simulink model "bal_main_alpha"  (R2015a)
settings: Solver=ode45  StartTime=0.0  StopTime=600  RelTol=1e-3
undefined symbols (not defined in the file): Alfa_zad, Cxa_Delta_1, Cxa_Delta_2, Cxa_Delta_3, Cxa_pol, Cya_Delta_1, Cya_Delta_2, Cya_Delta_3, Cya_pol, Delta_1_zad, Delta_2_zad, Delta_3_zad, h_zad, h_zad_D1_D2, h_zad_D3, mz_Alfa, mz_Delta_1, mz_Delta_2, mz_Delta_3, xt_zad
libraries: simulink x5
settings Model: Creator=Admin  LastModifiedBy=гена

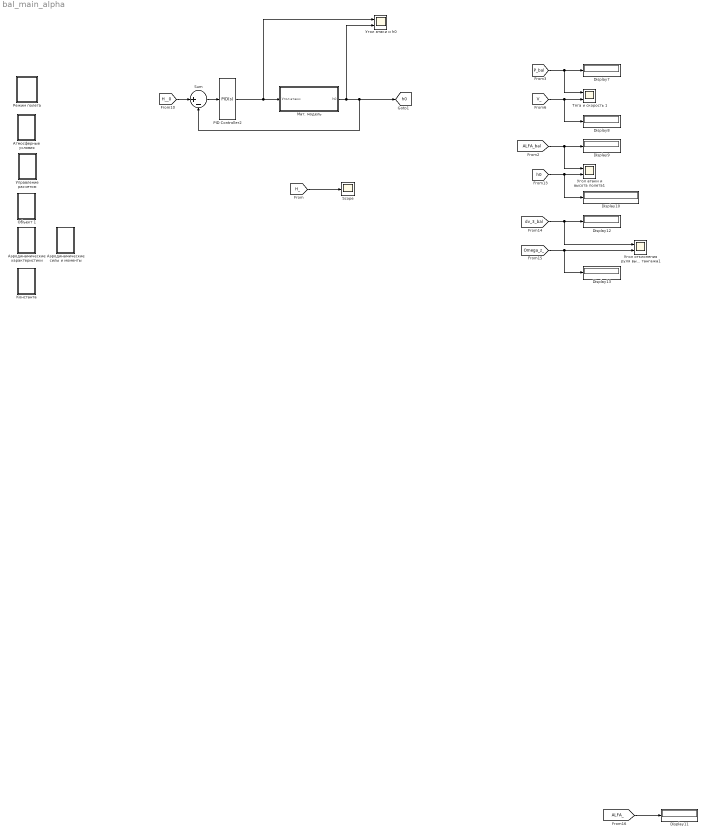
== system bal_main_alpha ==
  Display{7..13} (7 alike) : Display
  PID Controller2 : simulink/Continuous/PID Controller  Controller=PID  TimeDomain=Continuous-time  SampleTime=-1  IntegratorMethod=Forward Euler  FilterMethod=Forward Euler  Form=Parallel  UseFilter=on  ControllerParametersSource=internal  P=1.12  I=2  D=1  N=1  InitialConditionSource=internal  InitialConditionForIntegrator=0  InitialConditionForFilter=0  ExternalReset=none  LimitOutput=off  UpperSaturationLimit=inf  LowerSaturationLimit=-inf  LinearizeAsGain=on  AntiWindupMode=none  Kb=1  TrackingMode=off  Kt=1  PParamMin=[]  PParamMax=[]  IParamMin=[]  IParamMax=[]  DParamMin=[]  DParamMax=[]  NParamMin=[]  NParamMax=[]  KbParamMin=[]  KbParamMax=[]  KtParamMin=[]  KtParamMax=[]  POutMin=[]  POutMax=[]  IOutMin=[]  IOutMax=[]  DOutMin=[]  DOutMax=[]  NOutMin=[]  NOutMax=[]  KbOutMin=[]  KbOutMax=[]  KtOutMin=[]  KtOutMax=[]  IntegratorOutMin=[]  IntegratorOutMax=[]  FilterOutMin=[]  FilterOutMax=[]  SumOutMin=[]  SumOutMax=[]  SumI1OutMin=[]  SumI1OutMax=[]  SumI2OutMin=[]  SumI2OutMax=[]  SumI3OutMin=[]  SumI3OutMax=[]  SumDOutMin=[]  SumDOutMax=[]  SaturationOutMin=[]  SaturationOutMax=[]  IntegratorContinuousStateAttributes=''  IntegratorStateMustResolveToSignalObject=off  IntegratorRTWStateStorageClass=Auto  FilterContinuousStateAttributes=''  FilterStateMustResolveToSignalObject=off  FilterRTWStateStorageClass=Auto  DifferentiatorICPrevScaledInput=0  DifferentiatorOutMin=[]  DifferentiatorOutMax=[]
  Scope : Scope
  Sum : Sum  Inputs=|+-
  Атмосферные условия : Subsystem
  Аэродинамические характеристики : Subsystem
  Аэродинамические силы и моменты : Subsystem
  Константа : Subsystem
  Мат. модель : Subsystem
  Объект 1 : Subsystem
  Режим полета : Subsystem  mask(Параметры исходного полета){M_LA=1000, V_0=50, H_0=0.15}
      mask prompts: M_LA "Полетная масса, кг"; V_0 "Скорость полета, м/с"; H_0 "Высота полета, м"
  Тяга и скорость 1 : Scope  NumInputPorts=2
      settings: TimeRange=100  YMin=0~20  YMax=7000~55  SaveName=ScopeData3
  Угол атаки и высота полета1 : Scope  NumInputPorts=2
      settings: TimeRange=100  YMin=-5~-0.6000000000000001  YMax=20~0.2999999999999999  SaveName=ScopeData4
  Угол атаки и h0 : Scope  NumInputPorts=2
      settings: TimeRange=100  YMin=0~20  YMax=7000~55
  Угол отклонения руля высоты и угловая скорость тангажа1 : Scope  NumInputPorts=2
      settings: TimeRange=100  YMin=-6~-5  YMax=14~5  SaveName=ScopeData5
  Управление расчетом : Subsystem
  tag scope: h0=global
  wires:
  [P_bal] -> Display7/1, Тяга и скорость 1/1
  [V_] -> Display8/1, Тяга и скорость 1/2
  [ALFA_bal] -> Display9/1, Угол атаки и высота полета1/1
  [h0] -> Display10/1, Угол атаки и высота полета1/2
  [dv_3_bal] -> Display12/1, Угол отклонения руля высоты и угловая скорость тангажа1/1
  [Omega_z_] -> Display13/1, Угол отклонения руля высоты и угловая скорость тангажа1/2
  [ALFA_] -> Display11/1
  Sum/1 -> PID Controller2/1
  [H__0] -> Sum/1
  PID Controller2/1 -> Мат. модель/1(Угол атаки), Угол атаки и h0/1
  Мат. модель/1(h0) -> Угол атаки и h0/2, Sum/2, [h0]
  [H_] -> Scope/1

== system bal_main_alpha/Атмосферные условия ==
  Плотность : Constant  Value=1.225
  tag scope: Ro=global
  wires:
  Плотность/1 -> [Ro]

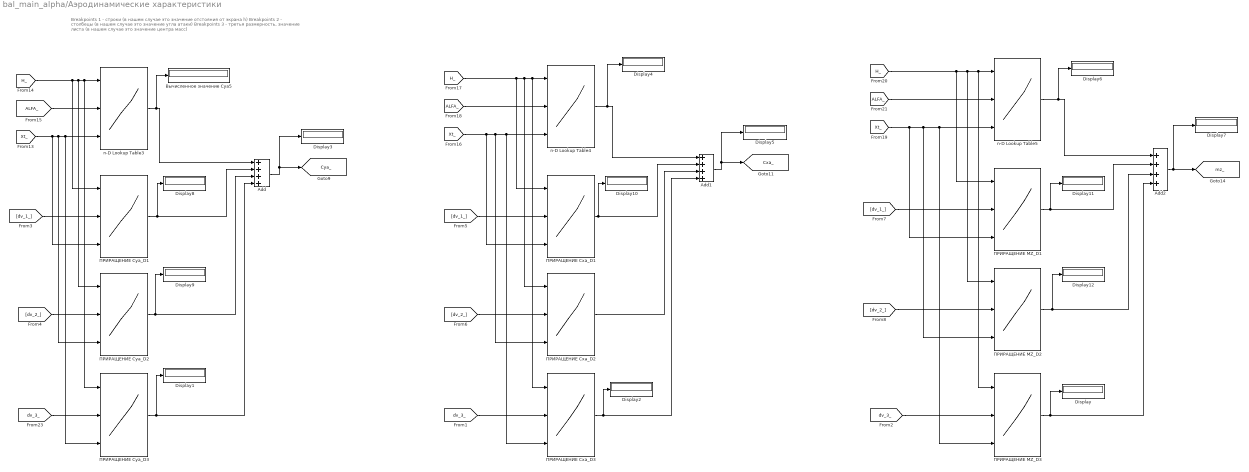
== system bal_main_alpha/Аэродинамические характеристики ==
  note: Breakpoints 1 - строки (в нашем случае это значение отстояния от экрана h)
      | Breakpoints 2 - столбецы (в нашем случае это значение угла атаки)
      | Breakpoints 3 - третья размерность, значение листа (в нашем случае это значение центра масс)
  Add : Sum  Inputs=++++
  Add1 : Sum  Inputs=++++
  Add2 : Sum  Inputs=++++
  Display{,1..12} (13 alike) : Display
  n-D Lookup Table3 : Lookup_n-D  NumberOfTableDimensions=3  BreakpointsForDimension1=h_zad  BreakpointsForDimension2=Alfa_zad  BreakpointsForDimension3=xt_zad  Table=Cya_pol  InternalRulePriority=Speed  RndMeth=Simplest  InputSameDT=on
  n-D Lookup Table4 : Lookup_n-D  NumberOfTableDimensions=3  BreakpointsForDimension1=h_zad  BreakpointsForDimension2=Alfa_zad  BreakpointsForDimension3=xt_zad  Table=Cxa_pol  InternalRulePriority=Speed  RndMeth=Simplest  InputSameDT=on
  n-D Lookup Table5 : Lookup_n-D  NumberOfTableDimensions=3  BreakpointsForDimension1=h_zad  BreakpointsForDimension2=Alfa_zad  BreakpointsForDimension3=xt_zad  Table=mz_Alfa  InternalRulePriority=Speed  RndMeth=Simplest  InputSameDT=on
  Вычисленное значение Суа5 : Display
  ПРИРАЩЕНИЕ Cxa_D1 : Lookup_n-D  NumberOfTableDimensions=3  BreakpointsForDimension1=h_zad_D1_D2  BreakpointsForDimension2=Delta_1_zad  BreakpointsForDimension3=xt_zad  Table=Cxa_Delta_1  InternalRulePriority=Speed  RndMeth=Simplest  InputSameDT=on
  ПРИРАЩЕНИЕ Cxa_D2 : Lookup_n-D  NumberOfTableDimensions=3  BreakpointsForDimension1=h_zad_D1_D2  BreakpointsForDimension2=Delta_2_zad  BreakpointsForDimension3=xt_zad  Table=Cxa_Delta_2  InternalRulePriority=Speed  RndMeth=Simplest  InputSameDT=on
  ПРИРАЩЕНИЕ Cxa_D3 : Lookup_n-D  NumberOfTableDimensions=3  BreakpointsForDimension1=h_zad_D3  BreakpointsForDimension2=Delta_3_zad  BreakpointsForDimension3=xt_zad  Table=Cxa_Delta_3  InternalRulePriority=Speed  RndMeth=Simplest  InputSameDT=on
  ПРИРАЩЕНИЕ Cya_D1 : Lookup_n-D  NumberOfTableDimensions=3  BreakpointsForDimension1=h_zad_D1_D2  BreakpointsForDimension2=Delta_1_zad  BreakpointsForDimension3=xt_zad  Table=Cya_Delta_1  InternalRulePriority=Speed  RndMeth=Simplest  InputSameDT=on
  ПРИРАЩЕНИЕ Cya_D2 : Lookup_n-D  NumberOfTableDimensions=3  BreakpointsForDimension1=h_zad_D1_D2  BreakpointsForDimension2=Delta_2_zad  BreakpointsForDimension3=xt_zad  Table=Cya_Delta_2  InternalRulePriority=Speed  RndMeth=Simplest  InputSameDT=on
  ПРИРАЩЕНИЕ Cya_D3 : Lookup_n-D  NumberOfTableDimensions=3  BreakpointsForDimension1=h_zad_D3  BreakpointsForDimension2=Delta_3_zad  BreakpointsForDimension3=xt_zad  Table=Cya_Delta_3  InternalRulePriority=Speed  RndMeth=Simplest  InputSameDT=on
  ПРИРАЩЕНИЕ MZ_D1 : Lookup_n-D  NumberOfTableDimensions=3  BreakpointsForDimension1=h_zad_D1_D2  BreakpointsForDimension2=Delta_1_zad  BreakpointsForDimension3=xt_zad  Table=mz_Delta_1  InternalRulePriority=Speed  RndMeth=Simplest  InputSameDT=on
  ПРИРАЩЕНИЕ MZ_D2 : Lookup_n-D  NumberOfTableDimensions=3  BreakpointsForDimension1=h_zad_D1_D2  BreakpointsForDimension2=Delta_2_zad  BreakpointsForDimension3=xt_zad  Table=mz_Delta_2  InternalRulePriority=Speed  RndMeth=Simplest  InputSameDT=on
  ПРИРАЩЕНИЕ MZ_D3 : Lookup_n-D  NumberOfTableDimensions=3  BreakpointsForDimension1=h_zad_D3  BreakpointsForDimension2=Delta_3_zad  BreakpointsForDimension3=xt_zad  Table=mz_Delta_3  InternalRulePriority=Speed  RndMeth=Simplest  InputSameDT=on
  tag scope: Cxa_=global, Cya_=global, mz_=global
  wires:
  [H_] -> ПРИРАЩЕНИЕ Cya_D3/1, n-D Lookup Table3/1, ПРИРАЩЕНИЕ Cya_D2/1, ПРИРАЩЕНИЕ Cya_D1/1
  [Xt_] -> ПРИРАЩЕНИЕ Cya_D2/3, ПРИРАЩЕНИЕ Cya_D3/3, n-D Lookup Table3/3, ПРИРАЩЕНИЕ Cya_D1/3
  n-D Lookup Table3/1 -> Вычисленное значение Суа5/1, Add/1
  [H_] -> ПРИРАЩЕНИЕ Cxa_D1/1, ПРИРАЩЕНИЕ Cxa_D2/1, ПРИРАЩЕНИЕ Cxa_D3/1, n-D Lookup Table4/1
  [Xt_] -> ПРИРАЩЕНИЕ Cxa_D1/3, ПРИРАЩЕНИЕ Cxa_D2/3, n-D Lookup Table4/3, ПРИРАЩЕНИЕ Cxa_D3/3
  [ALFA_] -> n-D Lookup Table5/2
  [ALFA_] -> n-D Lookup Table4/2
  [ALFA_] -> n-D Lookup Table3/2
  [Xt_] -> ПРИРАЩЕНИЕ MZ_D1/3, ПРИРАЩЕНИЕ MZ_D2/3, n-D Lookup Table5/3, ПРИРАЩЕНИЕ MZ_D3/3
  [dv_3_] -> ПРИРАЩЕНИЕ Cxa_D3/2
  Add/1 -> Display3/1, [Cya_]
  n-D Lookup Table4/1 -> Display4/1, Add1/1
  Add1/1 -> Display5/1, [Cxa_]
  n-D Lookup Table5/1 -> Display6/1, Add2/1
  Add2/1 -> Display7/1, [mz_]
  [dv_3_] -> ПРИРАЩЕНИЕ MZ_D3/2
  [dv_1_] -> ПРИРАЩЕНИЕ Cya_D1/2
  [dv_2_] -> ПРИРАЩЕНИЕ Cya_D2/2
  ПРИРАЩЕНИЕ Cya_D1/1 -> Display8/1, Add/2
  ПРИРАЩЕНИЕ Cya_D2/1 -> Display9/1, Add/3
  [dv_3_] -> ПРИРАЩЕНИЕ Cya_D3/2
  ПРИРАЩЕНИЕ Cya_D3/1 -> Display1/1, Add/4
  ПРИРАЩЕНИЕ Cxa_D3/1 -> Display2/1, Add1/4
  [dv_1_] -> ПРИРАЩЕНИЕ Cxa_D1/2
  ПРИРАЩЕНИЕ Cxa_D1/1 -> Display10/1, Add1/2
  [dv_2_] -> ПРИРАЩЕНИЕ Cxa_D2/2
  ПРИРАЩЕНИЕ Cxa_D2/1 -> Add1/3
  ПРИРАЩЕНИЕ MZ_D3/1 -> Display/1, Add2/4
  [dv_1_] -> ПРИРАЩЕНИЕ MZ_D1/2
  ПРИРАЩЕНИЕ MZ_D1/1 -> Display11/1, Add2/2
  [H_] -> ПРИРАЩЕНИЕ MZ_D2/1, ПРИРАЩЕНИЕ MZ_D3/1, n-D Lookup Table5/1, ПРИРАЩЕНИЕ MZ_D1/1
  [dv_2_] -> ПРИРАЩЕНИЕ MZ_D2/2
  ПРИРАЩЕНИЕ MZ_D2/1 -> Display12/1, Add2/3

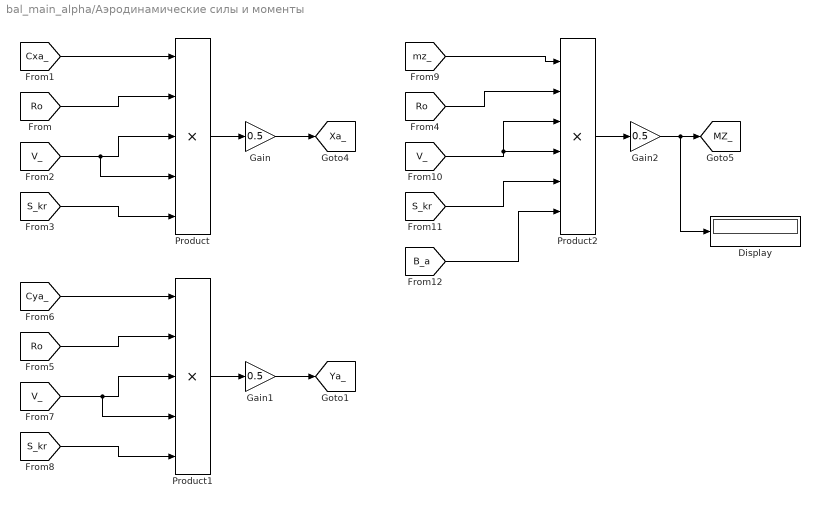
== system bal_main_alpha/Аэродинамические силы и моменты ==
  Display : Display
  Gain : Gain  Gain=0.5
  Gain1 : Gain  Gain=0.5
  Gain2 : Gain  Gain=0.5
  Product : Product  Inputs=*****
  Product1 : Product  Inputs=*****
  Product2 : Product  Inputs=******
  tag scope: MZ_=global, Xa_=global, Ya_=global
  wires:
  Product/1 -> Gain/1
  [S_kr] -> Product/5
  Gain/1 -> [Xa_]
  [Cxa_] -> Product/1
  [Ro] -> Product/2
  [V_] -> Product/4, Product/3
  Product1/1 -> Gain1/1
  [S_kr] -> Product1/5
  Gain1/1 -> [Ya_]
  [Cya_] -> Product1/1
  [Ro] -> Product1/2
  [V_] -> Product1/4, Product1/3
  Product2/1 -> Gain2/1
  [S_kr] -> Product2/5
  Gain2/1 -> Display/1, [MZ_]
  [mz_] -> Product2/1
  [Ro] -> Product2/2
  [B_a] -> Product2/6
  [V_] -> Product2/4, Product2/3

== system bal_main_alpha/Константа ==
  RAD : Constant  Value=57.3
  g : Constant  Value=9.81
  tag scope: RAD=global, g_=global
  wires:
  g/1 -> [g_]
  RAD/1 -> [RAD]

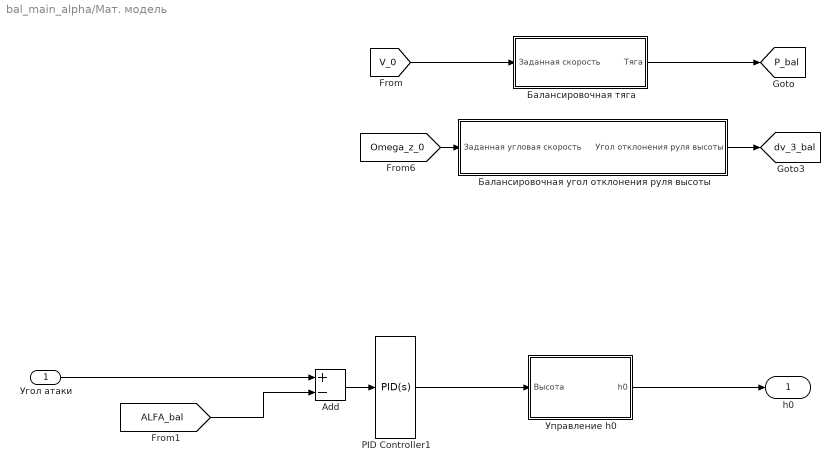
== system bal_main_alpha/Мат. модель ==
  Угол атаки : Inport
  Add : Sum  Inputs=+-
  PID Controller1 : simulink/Continuous/PID Controller  Controller=PID  TimeDomain=Continuous-time  SampleTime=-1  IntegratorMethod=Forward Euler  FilterMethod=Forward Euler  Form=Parallel  UseFilter=on  ControllerParametersSource=internal  P=0.0917439667717994  I=0.0166206189219194  D=-0.151733255398007  N=0.604639810377417  InitialConditionSource=internal  InitialConditionForIntegrator=0  InitialConditionForFilter=0  ExternalReset=none  LimitOutput=off  UpperSaturationLimit=inf  LowerSaturationLimit=-inf  LinearizeAsGain=on  AntiWindupMode=none  Kb=1  TrackingMode=off  Kt=1  PParamMin=[]  PParamMax=[]  IParamMin=[]  IParamMax=[]  DParamMin=[]  DParamMax=[]  NParamMin=[]  NParamMax=[]  KbParamMin=[]  KbParamMax=[]  KtParamMin=[]  KtParamMax=[]  POutMin=[]  POutMax=[]  IOutMin=[]  IOutMax=[]  DOutMin=[]  DOutMax=[]  NOutMin=[]  NOutMax=[]  KbOutMin=[]  KbOutMax=[]  KtOutMin=[]  KtOutMax=[]  IntegratorOutMin=[]  IntegratorOutMax=[]  FilterOutMin=[]  FilterOutMax=[]  SumOutMin=[]  SumOutMax=[]  SumI1OutMin=[]  SumI1OutMax=[]  SumI2OutMin=[]  SumI2OutMax=[]  SumI3OutMin=[]  SumI3OutMax=[]  SumDOutMin=[]  SumDOutMax=[]  SaturationOutMin=[]  SaturationOutMax=[]  IntegratorContinuousStateAttributes=''  IntegratorStateMustResolveToSignalObject=off  IntegratorRTWStateStorageClass=Auto  FilterContinuousStateAttributes=''  FilterStateMustResolveToSignalObject=off  FilterRTWStateStorageClass=Auto  DifferentiatorICPrevScaledInput=0  DifferentiatorOutMin=[]  DifferentiatorOutMax=[]
  Балансировочная угол отклонения руля высоты : Subsystem
  Балансировочная тяга : Subsystem
  Управление h0 : Subsystem
  h0 : Outport
  tag scope: P_bal=global, dv_3_bal=global
  wires:
  [V_0] -> Балансировочная тяга/1(Заданная скорость)
  [Omega_z_0] -> Балансировочная угол отклонения руля высоты/1(Заданная угловая скорость)
  Балансировочная угол отклонения руля высоты/1(Угол отклонения руля высоты) -> [dv_3_bal]
  Балансировочная тяга/1(Тяга) -> [P_bal]
  Add/1 -> PID Controller1/1
  Угол атаки/1 -> Add/1
  [ALFA_bal] -> Add/2
  PID Controller1/1 -> Управление h0/1(Высота)
  Управление h0/1(h0) -> h0/1

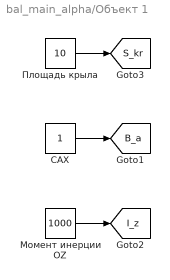
== system bal_main_alpha/Объект 1 ==
  Момент инерции ОZ : Constant  Value=1000
  Площадь крыла : Constant  Value=10
  САХ : Constant
  tag scope: B_a=global, I_z=global, S_kr=global
  wires:
  Площадь крыла/1 -> [S_kr]
  САХ/1 -> [B_a]
  Момент инерции ОZ/1 -> [I_z]

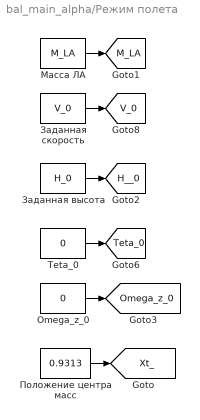
== system bal_main_alpha/Режим полета ==
  Omega_z_0 : Constant  Value=0
  Teta_0 : Constant  Value=0
  Заданная высота : Constant  Value=H_0
  Заданная скорость : Constant  Value=V_0
  Масса ЛА : Constant  Value=M_LA
  Положение центра масс : Constant  Value=0.9313
  tag scope: H__0=global, M_LA=global, Omega_z_0=global, Teta_0=global, V_0=global, Xt_=global
  wires:
  Заданная скорость/1 -> [V_0]
  Teta_0/1 -> [Teta_0]
  Масса ЛА/1 -> [M_LA]
  Заданная высота/1 -> [H__0]
  Omega_z_0/1 -> [Omega_z_0]
  Положение центра масс/1 -> [Xt_]

== system bal_main_alpha/Управление расчетом ==
  Условная начальная скорость : Constant  Value=50
  Условная начальная угловая скорость OZ : Constant  Value=0
  tag scope: OMEGA_Z_solve=global, V_solve=global
  wires:
  Условная начальная скорость/1 -> [V_solve]
  Условная начальная угловая скорость OZ/1 -> [OMEGA_Z_solve]

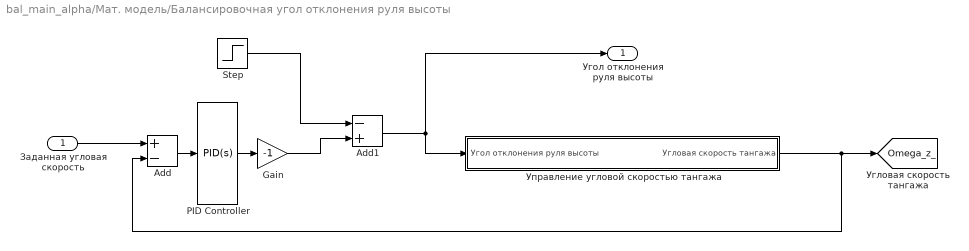
== system bal_main_alpha/Мат. модель/Балансировочная угол отклонения руля высоты ==
  Заданная угловая скорость : Inport
  Add : Sum  Inputs=+-
  Add1 : Sum  Inputs=-+
  Gain : Gain  Gain=-1
  PID Controller : simulink/Continuous/PID Controller  Controller=PID  TimeDomain=Continuous-time  SampleTime=-1  IntegratorMethod=Forward Euler  FilterMethod=Forward Euler  Form=Parallel  UseFilter=on  ControllerParametersSource=internal  P=0.379810440708384  I=0.0731035476397683  D=-0.0897634019475152  N=1.4222540202283  InitialConditionSource=internal  InitialConditionForIntegrator=0  InitialConditionForFilter=0  ExternalReset=none  LimitOutput=off  UpperSaturationLimit=inf  LowerSaturationLimit=-inf  LinearizeAsGain=on  AntiWindupMode=none  Kb=1  TrackingMode=off  Kt=1  PParamMin=[]  PParamMax=[]  IParamMin=[]  IParamMax=[]  DParamMin=[]  DParamMax=[]  NParamMin=[]  NParamMax=[]  KbParamMin=[]  KbParamMax=[]  KtParamMin=[]  KtParamMax=[]  POutMin=[]  POutMax=[]  IOutMin=[]  IOutMax=[]  DOutMin=[]  DOutMax=[]  NOutMin=[]  NOutMax=[]  KbOutMin=[]  KbOutMax=[]  KtOutMin=[]  KtOutMax=[]  IntegratorOutMin=[]  IntegratorOutMax=[]  FilterOutMin=[]  FilterOutMax=[]  SumOutMin=[]  SumOutMax=[]  SumI1OutMin=[]  SumI1OutMax=[]  SumI2OutMin=[]  SumI2OutMax=[]  SumI3OutMin=[]  SumI3OutMax=[]  SumDOutMin=[]  SumDOutMax=[]  SaturationOutMin=[]  SaturationOutMax=[]  IntegratorContinuousStateAttributes=''  IntegratorStateMustResolveToSignalObject=off  IntegratorRTWStateStorageClass=Auto  FilterContinuousStateAttributes=''  FilterStateMustResolveToSignalObject=off  FilterRTWStateStorageClass=Auto  DifferentiatorICPrevScaledInput=0  DifferentiatorOutMin=[]  DifferentiatorOutMax=[]
  Step : Step  Time=100  After=-10  SampleTime=0
  Управление угловой скоростью тангажа : Subsystem
  Угол отклонения руля высоты : Outport
  tag scope: Omega_z_=global
  wires:
  Add/1 -> PID Controller/1
  Заданная угловая скорость/1 -> Add/1
  Управление угловой скоростью тангажа/1(Угловая скорость тангажа) -> Add/2, [Omega_z_]
  PID Controller/1 -> Gain/1
  Step/1 -> Add1/1
  Gain/1 -> Add1/2
  Add1/1 -> Управление угловой скоростью тангажа/1(Угол отклонения руля высоты), Угол отклонения руля высоты/1

== system bal_main_alpha/Мат. модель/Балансировочная тяга ==
  Заданная скорость : Inport
  Add : Sum  Inputs=+-
  PID Controller : simulink/Continuous/PID Controller  Controller=PID  TimeDomain=Continuous-time  SampleTime=-1  IntegratorMethod=Forward Euler  FilterMethod=Forward Euler  Form=Parallel  UseFilter=on  ControllerParametersSource=internal  P=200  I=10  D=1  N=10  InitialConditionSource=internal  InitialConditionForIntegrator=0  InitialConditionForFilter=0  ExternalReset=none  LimitOutput=off  UpperSaturationLimit=inf  LowerSaturationLimit=-inf  LinearizeAsGain=on  AntiWindupMode=none  Kb=1  TrackingMode=off  Kt=1  PParamMin=[]  PParamMax=[]  IParamMin=[]  IParamMax=[]  DParamMin=[]  DParamMax=[]  NParamMin=[]  NParamMax=[]  KbParamMin=[]  KbParamMax=[]  KtParamMin=[]  KtParamMax=[]  POutMin=[]  POutMax=[]  IOutMin=[]  IOutMax=[]  DOutMin=[]  DOutMax=[]  NOutMin=[]  NOutMax=[]  KbOutMin=[]  KbOutMax=[]  KtOutMin=[]  KtOutMax=[]  IntegratorOutMin=[]  IntegratorOutMax=[]  FilterOutMin=[]  FilterOutMax=[]  SumOutMin=[]  SumOutMax=[]  SumI1OutMin=[]  SumI1OutMax=[]  SumI2OutMin=[]  SumI2OutMax=[]  SumI3OutMin=[]  SumI3OutMax=[]  SumDOutMin=[]  SumDOutMax=[]  SaturationOutMin=[]  SaturationOutMax=[]  IntegratorContinuousStateAttributes=''  IntegratorStateMustResolveToSignalObject=off  IntegratorRTWStateStorageClass=Auto  FilterContinuousStateAttributes=''  FilterStateMustResolveToSignalObject=off  FilterRTWStateStorageClass=Auto  DifferentiatorICPrevScaledInput=0  DifferentiatorOutMin=[]  DifferentiatorOutMax=[]
  Управление скоростью : Subsystem
  Тяга : Outport
  tag scope: V_=global
  wires:
  PID Controller/1 -> Тяга/1, Управление скоростью/1(Тяга)
  Add/1 -> PID Controller/1
  Заданная скорость/1 -> Add/1
  Управление скоростью/1(Скорость) -> Add/2, [V_]

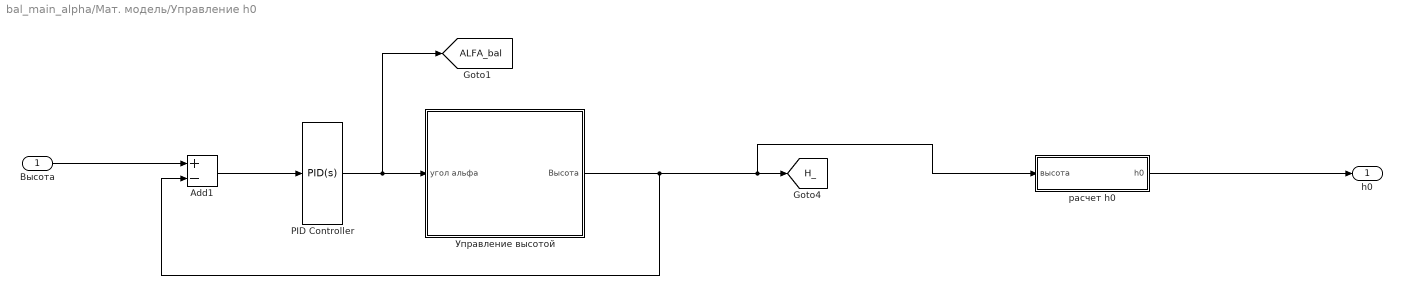
== system bal_main_alpha/Мат. модель/Управление h0 ==
  Высота : Inport
  Add1 : Sum  Inputs=+-
  PID Controller : simulink/Continuous/PID Controller  Controller=PID  TimeDomain=Continuous-time  SampleTime=-1  IntegratorMethod=Forward Euler  FilterMethod=Forward Euler  Form=Parallel  UseFilter=on  ControllerParametersSource=internal  P=10  I=10  D=10  N=10  InitialConditionSource=internal  InitialConditionForIntegrator=0  InitialConditionForFilter=0  ExternalReset=none  LimitOutput=off  UpperSaturationLimit=inf  LowerSaturationLimit=-inf  LinearizeAsGain=on  AntiWindupMode=none  Kb=1  TrackingMode=off  Kt=1  PParamMin=[]  PParamMax=[]  IParamMin=[]  IParamMax=[]  DParamMin=[]  DParamMax=[]  NParamMin=[]  NParamMax=[]  KbParamMin=[]  KbParamMax=[]  KtParamMin=[]  KtParamMax=[]  POutMin=[]  POutMax=[]  IOutMin=[]  IOutMax=[]  DOutMin=[]  DOutMax=[]  NOutMin=[]  NOutMax=[]  KbOutMin=[]  KbOutMax=[]  KtOutMin=[]  KtOutMax=[]  IntegratorOutMin=[]  IntegratorOutMax=[]  FilterOutMin=[]  FilterOutMax=[]  SumOutMin=[]  SumOutMax=[]  SumI1OutMin=[]  SumI1OutMax=[]  SumI2OutMin=[]  SumI2OutMax=[]  SumI3OutMin=[]  SumI3OutMax=[]  SumDOutMin=[]  SumDOutMax=[]  SaturationOutMin=[]  SaturationOutMax=[]  IntegratorContinuousStateAttributes=''  IntegratorStateMustResolveToSignalObject=off  IntegratorRTWStateStorageClass=Auto  FilterContinuousStateAttributes=''  FilterStateMustResolveToSignalObject=off  FilterRTWStateStorageClass=Auto  DifferentiatorICPrevScaledInput=0  DifferentiatorOutMin=[]  DifferentiatorOutMax=[]
  Управление высотой : Subsystem
  расчет h0 : Subsystem
  h0 : Outport
  tag scope: ALFA_bal=global, H_=global
  wires:
  расчет h0/1(h0) -> h0/1
  Высота/1 -> Add1/1
  Управление высотой/1(Высота) -> Add1/2, расчет h0/1(высота), [H_]
  PID Controller/1 -> [ALFA_bal], Управление высотой/1(угол альфа)
  Add1/1 -> PID Controller/1

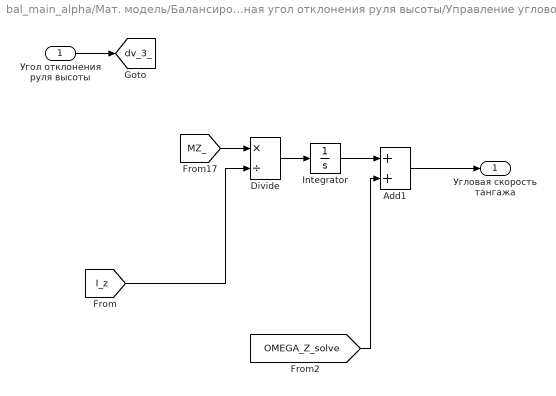
== system bal_main_alpha/Мат. модель/Балансировочная угол отклонения руля высоты/Управление угловой скоростью тангажа ==
  Угол отклонения руля высоты : Inport
  Add1 : Sum
  Divide : Product  Inputs=*/
  Integrator : Integrator
  Угловая скорость тангажа : Outport
  tag scope: dv_3_=global
  wires:
  Угол отклонения руля высоты/1 -> [dv_3_]
  [MZ_] -> Divide/1
  [I_z] -> Divide/2
  Divide/1 -> Integrator/1
  Integrator/1 -> Add1/1
  [OMEGA_Z_solve] -> Add1/2
  Add1/1 -> Угловая скорость тангажа/1

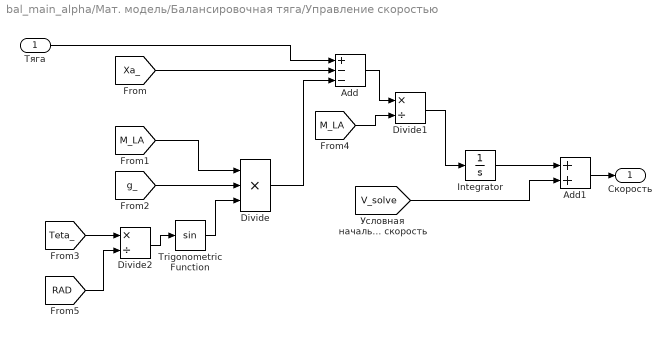
== system bal_main_alpha/Мат. модель/Балансировочная тяга/Управление скоростью ==
  Тяга : Inport
  Add : Sum  Inputs=+--
  Add1 : Sum
  Divide : Product  Inputs=***
  Divide1 : Product  Inputs=*/
  Divide2 : Product  Inputs=*/
  Integrator : Integrator
  Trigonometric Function : Trigonometry
  Скорость : Outport
  wires:
  [Xa_] -> Add/2
  Тяга/1 -> Add/1
  [M_LA] -> Divide1/2
  Divide/1 -> Add/3
  Divide1/1 -> Integrator/1
  [M_LA] -> Divide/1
  Trigonometric Function/1 -> Divide/3
  [g_] -> Divide/2
  Add/1 -> Divide1/1
  Add1/1 -> Скорость/1
  Integrator/1 -> Add1/1
  [V_solve] -> Add1/2
  [Teta_] -> Divide2/1
  Divide2/1 -> Trigonometric Function/1
  [RAD] -> Divide2/2

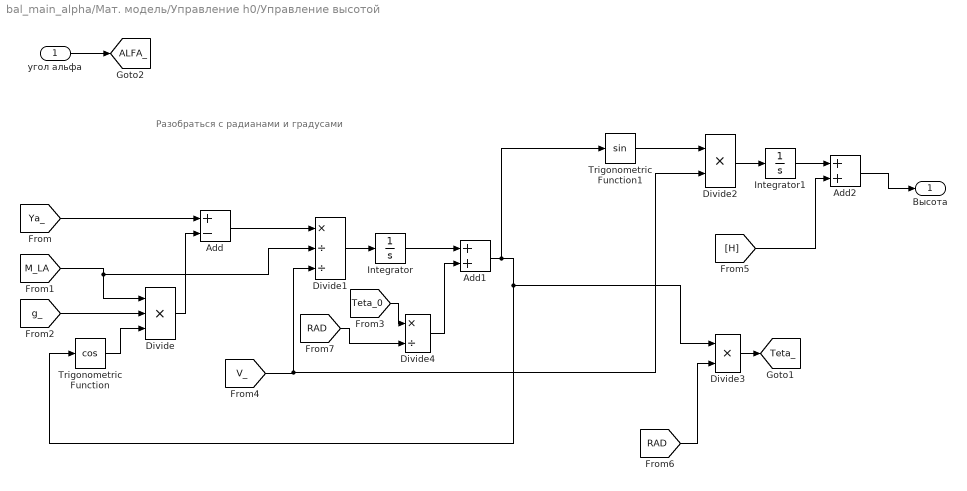
== system bal_main_alpha/Мат. модель/Управление h0/Управление высотой ==
  note: Разобраться с радианами и градусами
  угол альфа : Inport
  Add : Sum  Inputs=+-
  Add1 : Sum
  Add2 : Sum
  Divide : Product  Inputs=***
  Divide1 : Product  Inputs=*//
  Divide2 : Product  Inputs=**
  Divide3 : Product  Inputs=**
  Divide4 : Product  Inputs=*/
  Integrator : Integrator
  Integrator1 : Integrator
  Trigonometric Function : Trigonometry  Operator=cos
  Trigonometric Function1 : Trigonometry
  Высота : Outport
  tag scope: ALFA_=global, Teta_=global
  wires:
  [M_LA] -> Divide1/2, Divide/1
  Trigonometric Function/1 -> Divide/3
  [g_] -> Divide/2
  [Ya_] -> Add/1
  Divide/1 -> Add/2
  Add/1 -> Divide1/1
  [V_] -> Divide1/3, Divide2/2
  Divide1/1 -> Integrator/1
  Integrator/1 -> Add1/1
  Add1/1 -> Trigonometric Function/1, Divide3/1, Trigonometric Function1/1
  Trigonometric Function1/1 -> Divide2/1
  Divide2/1 -> Integrator1/1
  Integrator1/1 -> Add2/1
  [H] -> Add2/2
  Add2/1 -> Высота/1
  Divide3/1 -> [Teta_]
  [RAD] -> Divide3/2
  [Teta_0] -> Divide4/1
  Divide4/1 -> Add1/2
  [RAD] -> Divide4/2
  угол альфа/1 -> [ALFA_]

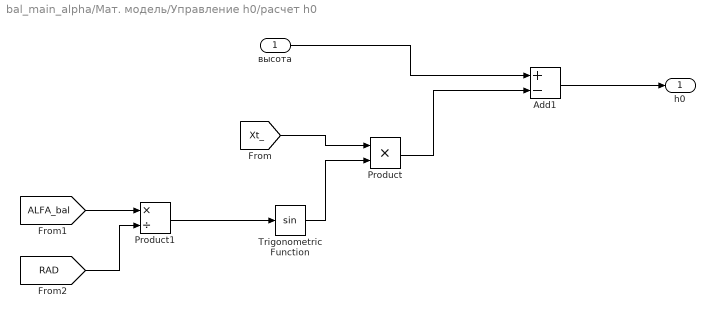
== system bal_main_alpha/Мат. модель/Управление h0/расчет h0 ==
  высота : Inport
  Add1 : Sum  Inputs=+-
  Product : Product
  Product1 : Product  Inputs=*/
  Trigonometric Function : Trigonometry
  h0 : Outport
  wires:
  Add1/1 -> h0/1
  Product/1 -> Add1/2
  [Xt_] -> Product/1
  Trigonometric Function/1 -> Product/2
  [ALFA_bal] -> Product1/1
  [RAD] -> Product1/2
  Product1/1 -> Trigonometric Function/1
  высота/1 -> Add1/1
